simulink model "p_d_control"  (R2015a)
settings: Solver=ode45  StartTime=0.0  StopTime=10.0  RelTol=1e-3
undefined symbols (not defined in the file): omega, zeta
settings Model: Creator=shohei  LastModifiedBy=shohei

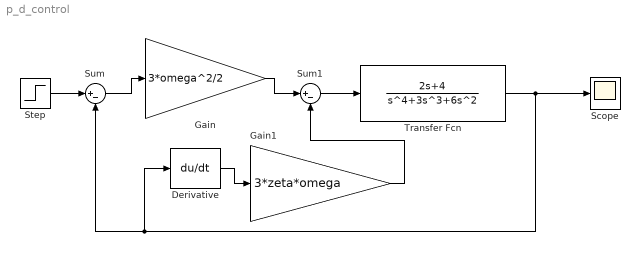
== system p_d_control ==
  Derivative : Derivative
  Gain : Gain  Gain=3*omega^2/2
  Gain1 : Gain  Gain=3*zeta*omega
  Scope : Scope
  Step : Step  SampleTime=0
  Sum : Sum  Inputs=|+-
  Sum1 : Sum  Inputs=|+-
  Transfer Fcn : TransferFcn  Numerator=[2 4]  Denominator=[1 3 6 0 0]
  wires:
  Transfer Fcn/1 -> Derivative/1, Sum/2, Scope/1
  Step/1 -> Sum/1
  Sum/1 -> Gain/1
  Gain/1 -> Sum1/1
  Sum1/1 -> Transfer Fcn/1
  Gain1/1 -> Sum1/2
  Derivative/1 -> Gain1/1
